simulink model "ICARO_III_debug_telemetry"  (R2014a)
settings: Solver=FixedStepDiscrete  StartTime=0.0  StopTime=inf  FixedStep=0.01  MaxStep=0.01  RelTol=1e-3
settings Model: Creator=regular  LastModifiedBy=ivald
settings DataIOCC: SignalLoggingSaveFormat=ModelDataLogs  SaveOutput=off  SaveTime=off
settings OptimizationCC: ExpressionDepthLimit=2147483647  OptimizeModelRefInitCode=on  LifeSpan=1
settings DebuggingCC: UnderspecifiedInitializationDetection=Classic  FcnCallInpInsideContextMsg=UseLocalSettings  StateNameClashWarn=warning
settings HardwareCC: ProdBitPerChar=16  ProdBitPerInt=16  ProdBitPerPointer=16  ProdLargestAtomicInteger=Integer  ProdIntDivRoundTo=Zero  ProdEndianess=LittleEndian  ProdWordSize=16  ProdHWDeviceType=Texas Instruments->C2000
settings SFSimCC: SimParseCustomCode=off
settings RTWCC: SystemTargetFile=idelink_ert.tlc  GenerateMakefile=off  TemplateMakefile=idelink_ert.tmf  Description=IDE Link ERT  ProcessScript=idelink_ert_make_rtw_hook
settings CodeAppCC: IgnoreCustomStorageClasses=off  CustomSymbolStrType=$N$R$M  InternalIdentifier=Classic
settings TargetHardwareResources: Description=Target Hardware Resources Component

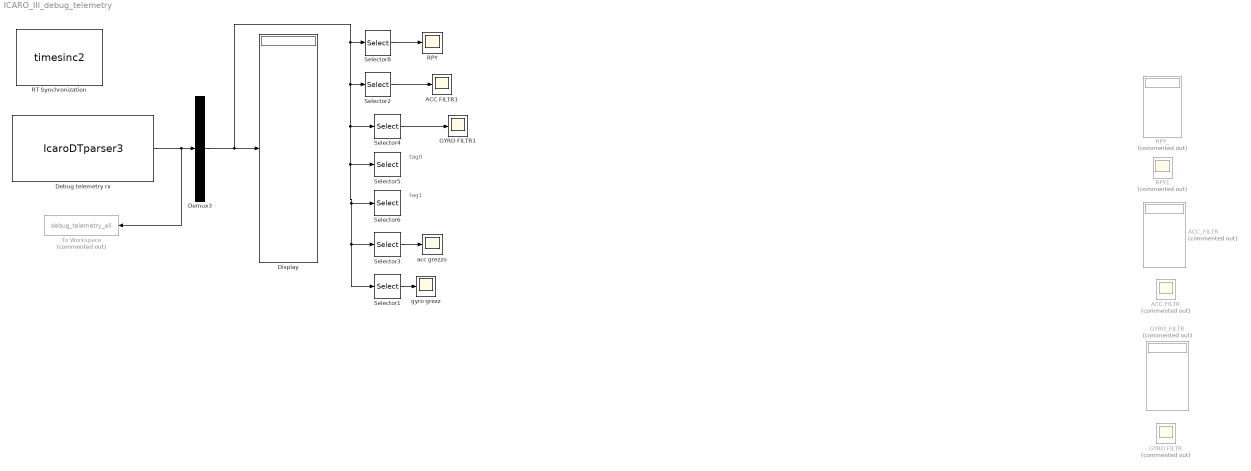
== system ICARO_III_debug_telemetry ==
  note: tag1
  note: tag0
  ACC FILTR : Scope  Commented=on
      settings: YMin=-16  SaveName=ScopeData4
  ACC FILTR1 : Scope
      settings: YMin=-16  SaveName=ScopeData6
  ACC_FILTR : Display  Commented=on
  Debug telemetry rx : S-Function  FunctionName=IcaroDTparser3  Parameters=ST, port_name,port_baud, float_num, blocking, outputtype  EnableBusSupport=off  mask{ST=1/100, port_name=3, float_num=30, port_baud=115200, blocking=0, outputtype=1}
      mask prompts: ST "Sample Time"; port_name "Com port number (int)"; float_num "Number of floats / bytes"; port_baud "Com port Baud rate"; blocking "blocking mode (0: non blocking ) (1:blocking w/ timeout)"; outputtype "output type (1: float, 0 bytes)"
      mask Display: disp('ICARO II \n Debug Telemetry RX');
  Demux3 : Demux  Outputs=1
  Display : Display
  GYRO FILTR : Scope  Commented=on
      settings: YMin=-16  SaveName=ScopeData2
  GYRO FILTR1 : Scope
      settings: YMin=-16  SaveName=ScopeData7
  GYRO_FILTR : Display  Commented=on
  RPY : Scope
      settings: YMin=-2  YMax=2
  RPY1 : Scope  Commented=on
      settings: YMin=-2  YMax=2  SaveName=ScopeData5
  RPY_ : Display  Commented=on
  RT Synchronization : S-Function  FunctionName=timesinc2  Parameters=st mf  EnableBusSupport=off  mask(Pseudo-Real Time synchronization for Simulink Schemes){st=0.01, mf=1}
      mask prompts: st "Sample Time"; mf "Multiply factor"
      mask help:
      | This block synchronizes Simulink Simulation with RealTime.
      | The Real-Time versus Simulation-Time alignment is done every "Sample Time" seconds.
      | The Multiply Factor accelerates or slows real-Time: Multiply Factor=1 means real-time, Multiply Factor=2 means two times faster than real-time.
      | Use a Multiply Factor strictly > 0!!
      mask Display: disp(sprintf('RT Synchronization\n\nSample Time: %f\n Accelerator: %f',st,mf));
  Selector1 : Selector  InputPortWidth=22  Indices=[20:22]
  Selector2 : Selector  InputPortWidth=22  Indices=[5:7]
  Selector3 : Selector  InputPortWidth=22  Indices=[17:19]
  Selector4 : Selector  InputPortWidth=22  Indices=[8:10]
  Selector5 : Selector  InputPortWidth=22  Indices=[11:13]
  Selector6 : Selector  InputPortWidth=22  Indices=[14:16]
  Selector8 : Selector  InputPortWidth=22  Indices=[2:4]
  To Workspace : ToWorkspace  Commented=on  VariableName=debug_telemetry_all  SampleTime=-1
  acc grezzo : Scope
      settings: YMin=-15  YMax=2  SaveName=ScopeData3
  "gyro grezz " : Scope
      settings: YMin=-1  YMax=1
  wires:
  Debug telemetry rx/1 -> To Workspace/1, Demux3/1
  Demux3/1 -> Selector2/1, Selector4/1, Selector5/1, Selector1/1, Selector3/1, Selector6/1, Selector8/1, Display/1
  Selector8/1 -> RPY/1
  Selector1/1 -> "gyro grezz "/1
  Selector3/1 -> acc grezzo/1
  ? -> GYRO FILTR/1, GYRO_FILTR/1
  ? -> ACC_FILTR/1, ACC FILTR/1
  Selector2/1 -> ACC FILTR1/1
  Selector4/1 -> GYRO FILTR1/1
  ? -> RPY_/1, RPY1/1
